simulink model "Esercitazione_Branz"  (R2023b)
settings: Solver=VariableStepAuto  StartTime=0.0  StopTime=tf  RelTol=1e-3
values from neighbouring files (symbols this model uses):
  a = [a1 a2 a3 a4]    [init.m]
  pf = [-1.6 0.9 180]'    [scenario_data.m]
settings Model: Creator=franc  LastModifiedBy=franc

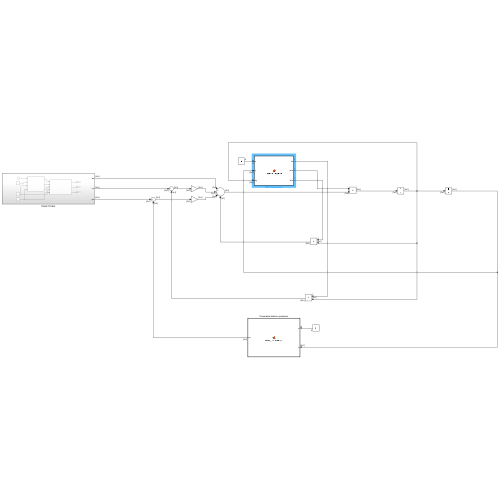
[thumbnail: Simulink's stored preview of the top-level diagram]
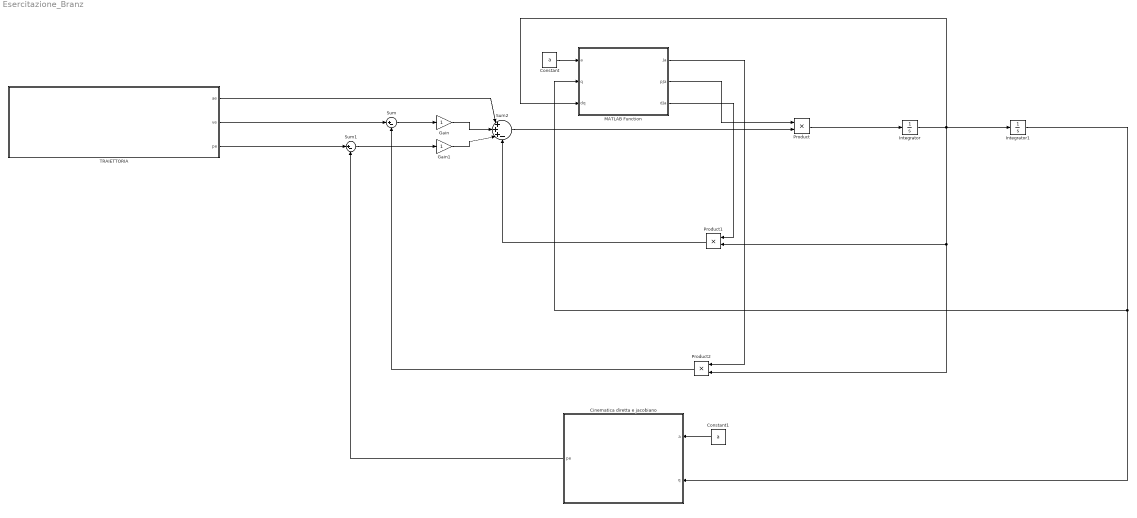
== system Esercitazione_Branz ==
  Cinematica diretta e jacobiano : MATLAB Function  TreatAsAtomicUnit=on
  Constant : Constant  Value=a
  Constant1 : Constant  Value=a
  Gain : Gain
  Gain1 : Gain
  Integrator : Integrator
  Integrator1 : Integrator
  MATLAB Function : MATLAB Function  TreatAsAtomicUnit=on
  Product : Product
  Product1 : Product
  Product2 : Product
  Sum : Sum  Inputs=|+-
  Sum1 : Sum  Inputs=|+-
  Sum2 : Sum  Inputs=|+++-
  TRAIETTORIA : Subsystem
  wires:
  Product/1 -> Integrator/1
  TRAIETTORIA/1(ae) -> Sum2/1
  TRAIETTORIA/2(ve) -> Sum/1
  Gain1/1 -> Sum2/3
  TRAIETTORIA/3(pe) -> Sum1/1
  Integrator1/1 -> Cinematica diretta e jacobiano/2(q), MATLAB Function/2(q)
  Sum2/1 -> Product/2
  Constant1/1 -> Cinematica diretta e jacobiano/1(a)
  Constant/1 -> MATLAB Function/1(a)
  Cinematica diretta e jacobiano/1(pe) -> Sum1/2
  MATLAB Function/3(dJa) -> Product1/1
  MATLAB Function/2(pJa) -> Product/1
  MATLAB Function/1(Ja) -> Product2/1
  Sum1/1 -> Gain1/1
  Product2/1 -> Sum/2
  Product1/1 -> Sum2/4
  Sum/1 -> Gain/1
  Gain/1 -> Sum2/2
  Integrator/1 -> Product1/2, Product2/2, MATLAB Function/3(dq), Integrator1/1

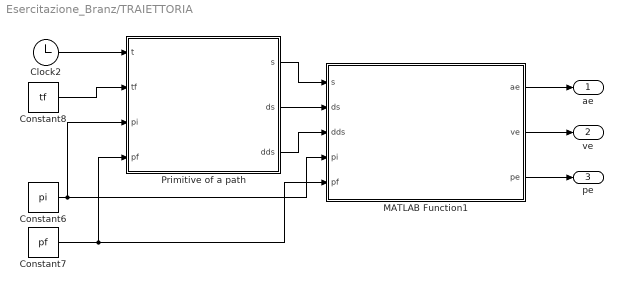
== system Esercitazione_Branz/TRAIETTORIA ==
  Clock2 : Clock
  Constant6 : Constant  Value=pi
  Constant7 : Constant  Value=pf
  Constant8 : Constant  Value=tf
  MATLAB Function1 : MATLAB Function  TreatAsAtomicUnit=on
  Primitive of a path : MATLAB Function  TreatAsAtomicUnit=on
  ae : Outport
  ve : Outport  Port=2
  pe : Outport  Port=3
  wires:
  Clock2/1 -> Primitive of a path/1(t)
  Primitive of a path/1(s) -> MATLAB Function1/1(s)
  Constant7/1 -> MATLAB Function1/5(pf), Primitive of a path/4(pf)
  Constant6/1 -> MATLAB Function1/4(pi), Primitive of a path/3(pi)
  Primitive of a path/3(dds) -> MATLAB Function1/3(dds)
  Primitive of a path/2(ds) -> MATLAB Function1/2(ds)
  Constant8/1 -> Primitive of a path/2(tf)
  MATLAB Function1/3(pe) -> pe/1
  MATLAB Function1/1(ae) -> ae/1
  MATLAB Function1/2(ve) -> ve/1

== matlab function Esercitazione_Branz/Cinematica diretta e jacobiano ==
  data: a input; q input; pe output
function pe = direct_kinematics(a,q)

% Numero di gradi di libertà del manipolatore
n = length(a);

% Vettore delle varibili di giunto in radianti
q = deg2rad(q);

% Applicazione delle ipotesi per gli elementi della tabella DH
d = zeros(n);
alpha = zeros(n);

% Calcolo delle matrici di trasformazione
A = zeros(4,4);
Tn0 = eye(4);
p = zeros(3,n+1);
for i = 1:n
    % Matrice di trasformazione per il giunto i-esimo
    A(1,1) = cos(q(i));
    A(1,2) = -sin(q(i))*cos(alpha(i));
    A(1,3) = sin(q(i))*sin(alpha(i));
    A(1,4) = a(i)*cos(q(i));

    A(2,1) = sin(q(i));
    A(2,2) = cos(q(i))*cos(alpha(i));
    A(2,3) = -cos(q(i))*sin(alpha(i));
    A(2,4) = a(i)*sin(q(i));

    A(3,1) = 0;
    A(3,2) = sin(alpha(i));
    A(3,3) = cos(alpha(i));
    A(3,4) = d(i);

    A(4,1:end-1) = 0;
    A(4,end) = 1;

    % Moltiplicazione delle matrici di trasformazione
    Tn0 = Tn0*A;
    
    % Calcolo del vettore di traslazione dell'end effector rispetto al
    % giunto i
    p(:,i+1) = Tn0(1:3,4);
end

% Calcolo matrice di trasferimento da base a 0
T0b = eye(4);
% Calcolo matrice di trasferimento da n ad end effector
Ten = [0 0 1 0; 0 1 0 0; 1 0 0 0; 0 0 0 1];
% Calcolo matrice di trasformazione dal sistema di riferimento base a
% quello dell'end effector
Teb = T0b*Tn0*Ten;
% Calcolo del vettore di posa dell'end effector
pe = Teb(1:3,4);

% % Calcolo del versore z 
% z = [0 0 1]';
% % Calcolo dello Jacobiano geometrico
% J = zeros(6,4);
% for i = 1:n
%     J(1:3,i) = cross(z,(pe-p(:,i)));
%     J(4:end,i) = z;
% end
% 
% % Ridefinizione dello jacobiano a rango pieno
% Jrk = zeros(3,4);
% Jrk(1:2,:) = J(1:2,:);
% Jrk(3,:) = J(6,:);
% 
% % Calcolo dello jacobiano pseudoinverso
% Jp = pinv(Jrk); 
%

== matlab function Esercitazione_Branz/MATLAB Function ==
  data: a input; Ja output; q input; dq input; pJa output; dJa output
function [Ja,pJa,dJa] = analytic_jacobian(a,q,dq)

% Function che implementa lo jacobiano analitico
% Input:  - a = [a1 a2 a3 a4] vettore delle lunghezze dei link
%         - q = [q1 q2 q3 q4] vettore delle variabili di giunto
% Output: - Ja = [3x4]

% Conversione in radianti delle variabili di giunto 
q = deg2rad(q);
% Calcolo dello jacobiano analitico
Ja = zeros(3,4);

Ja(1,1) = -a(1)*sin(q(1))-a(2)*sin(q(1)+q(2))-a(3)*sin(q(1)+q(2)+q(3)) ...
    -a(4)*sin(q(1)+q(2)+q(3)+q(4));
Ja(1,2) = -a(2)*sin(q(1)+q(2))-a(3)*sin(q(1)+q(2)+q(3)) ...
    -a(4)*sin(q(1)+q(2)+q(3)+q(4));
Ja(1,3) = -a(3)*sin(q(1)+q(2)+q(3))-a(4)*sin(q(1)+q(2)+q(3)+q(4));
Ja(1,4) = -a(4)*sin(q(1)+q(2)+q(3)+q(4));

Ja(2,1) = a(1)*cos(q(1))+a(2)*cos(q(1)+q(2))+a(3)*cos(q(1)+q(2)+q(3))...
    +a(4)*cos(q(1)+q(2)+q(3)+q(4));
Ja(2,2) = a(2)*cos(q(1)+q(2))+a(3)*cos(q(1)+q(2)+q(3))...
    +a(4)*cos(q(1)+q(2)+q(3)+q(4));
Ja(2,3) = a(3)*cos(q(1)+q(2)+q(3))+a(4)*cos(q(1)+q(2)+q(3)+q(4));
Ja(2,4) = a(4)*cos(q(1)+q(2)+q(3)+q(4));

Ja(3,:) = 1;

% Calcolo della matrice pseudoinversa dello jacobiano
pJa = pinv(Ja);

% Calcolo della derivata dello jacobiano
dJa = zeros(3,4);

dJa(1,1) = -a(1)*cos(q(1))*dq(1)-a(2)*cos(q(1)+q(2))*(dq(1)+dq(2)) ...
    -a(3)*cos(q(1)+q(2)+q(3))*(dq(1)+dq(2)+dq(3)) ...
    -a(4)*cos(q(1)+q(2)+q(3)+q(4))*(dq(1)+dq(2)+dq(3)+dq(4));
dJa(1,2) = -a(2)*cos(q(1)+q(2))*(dq(1)+dq(2)) ...
    -a(3)*cos(q(1)+q(2)+q(3))*(dq(1)+dq(2)+dq(3)) ...
    -a(4)*cos(q(1)+q(2)+q(3)+q(4))*(dq(1)+dq(2)+dq(3)+dq(4));
dJa(1,3) = -a(3)*cos(q(1)+q(2)+q(3))*(dq(1)+dq(2)+dq(3)) ...
    -a(4)*cos(q(1)+q(2)+q(3)+q(4))*(dq(1)+dq(2)+dq(3)+dq(4));
dJa(1,4) = -a(4)*cos(q(1)+q(2)+q(3)+q(4))*(dq(1)+dq(2)+dq(3)+dq(4));

dJa(2,1) = -a(1)*sin(q(1))*dq(1)-a(2)*sin(q(1)+q(2))*(dq(1)+dq(2)) ...
    -a(3)*sin(q(1)+q(2)+q(3))*(dq(1)+dq(2)+dq(3))...
    -a(4)*sin(q(1)+q(2)+q(3)+q(4))*(dq(1)+dq(2)+dq(3)+dq(4));
dJa(2,2) = -a(2)*sin(q(1)+q(2))*(dq(1)+dq(2)) ...
    -a(3)*sin(q(1)+q(2)+q(3))*(dq(1)+dq(2)+dq(3))...
    -a(4)*sin(q(1)+q(2)+q(3)+q(4))*(dq(1)+dq(2)+dq(3)+dq(4));
dJa(2,3) = -a(3)*sin(q(1)+q(2)+q(3))*(dq(1)+dq(2)+dq(3))...
    -a(4)*sin(q(1)+q(2)+q(3)+q(4))*(dq(1)+dq(2)+dq(3)+dq(4));
dJa(2,4) = -a(4)*sin(q(1)+q(2)+q(3)+q(4))*(dq(1)+dq(2)+dq(3)+dq(4));

dJa(3,:) = 0;

== matlab function Esercitazione_Branz/TRAIETTORIA/MATLAB Function1 ==
  data: ae output; ve output; s input; pe output; ds input; dds input; pi input; pf input
function [ae,ve,pe] = rectilinar_tajectory(s,ds,dds,pi,pf)

d = norm(pf(1:2)-pi(1:2));

% Rappresentazione parametrica della traiettoria
pe = pi+s/d*(pf-pi);
ve = ds/d*(pf-pi);
ae = dds/d*(pf-pi);

== matlab function Esercitazione_Branz/TRAIETTORIA/Primitive of a path ==
  data: t input; s output; tf input; pi input; pf input; ds output; dds output
function [s,ds,dds] = path_primitive(t,tf,pi,pf)

% Distanza tra la posizione iniziale e la posizione finale dell'end
% effector
d = norm(pf(1:2)-pi(1:2));

% Polinomio di quinto grado e le sue derivate:
% s = x5*t_f^5+x4*t_f^4+x3*t_f^3+x2*t_f^2+x1*t_f+x0;
% s_dot = 5*x5*t_f^4+4*x4*t_f^3+3*x3*t_f^2+2*x2*t_f+x1;
% s_2dot = 4*5*x5*t_f^3+3*4*x4*t_f^2+2*3*x3*t_f+2*x2;
% Condizioni sul tempo iniziale:
% s(0) = 0;
% s_dot(0) = 0;
% s_2dot(0) = 0;
% Condizioni sul tempo finale:
% s(t_f) = d;
% s_dot(t_f) = 0;
% s_2dot(t_f) = 0;

% Calcolo dei coefficienti del polinomio 
A = [0 0 0 0 0 1;
     tf^5 tf^4 tf^3 tf^2 tf 1;
     0 0 0 0 1 0;
     5*tf^4 4*tf^3 3*tf^2 2*tf 1 0;
     0 0 0 2 0 0;
     20*tf^3 12*tf^2 6*tf 2 0 0];
b = [0 d 0 0 0 0]';
coeff = A\b;

% Rappresentazione parametrica del path e delle sue derivate
s = coeff(1)*t^5+coeff(2)*t^4+coeff(3)*t^3+coeff(4)*t^2+coeff(5)*t+coeff(6);
ds = 5*coeff(1)*t^4+4*coeff(2)*t^3+3*coeff(3)*t^2+2*coeff(4)*t^1+coeff(5);
dds = 20*coeff(1)*t^3+12*coeff(2)*t^2+6*coeff(3)*t^1+2*coeff(4);
